simulink model "maglev_linear_model"  (R2021a)
settings: Solver=VariableStepAuto  StartTime=0.0  StopTime=0.2  RelTol=1e-3
settings Model: Creator=user  LastModifiedBy=user

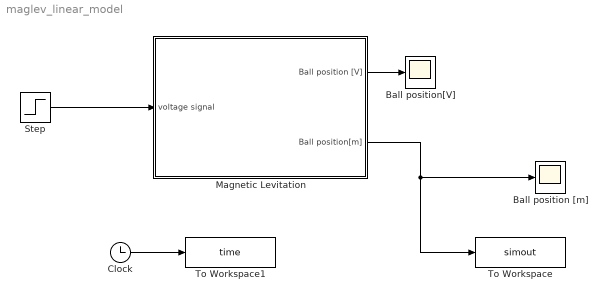
== system maglev_linear_model ==
  Ball position [m] : Scope
  Ball position[V] : Scope
  Clock : Clock
  Magnetic Levitation : Subsystem
  Step : Step  SampleTime=0
  To Workspace : ToWorkspace  VariableName=simout  SampleTime=-1
      settings: Save2DSignal=2-D array (concatenate along first dimension)
  To Workspace1 : ToWorkspace  VariableName=time  SampleTime=0.01
      settings: Save2DSignal=2-D array (concatenate along first dimension)
  wires:
  Step/1 -> Magnetic Levitation/1(voltage signal)
  Magnetic Levitation/2(Ball position[m]) -> To Workspace/1, Ball position [m]/1
  Magnetic Levitation/1(Ball position [V]) -> Ball position[V]/1
  Clock/1 -> To Workspace1/1

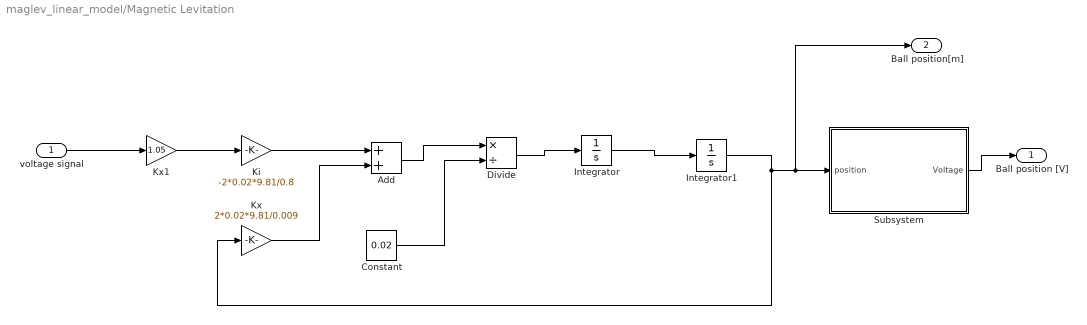
== system maglev_linear_model/Magnetic Levitation ==
  voltage signal : Inport
  Add : Sum
  Constant : Constant  Value=0.02
  Divide : Product  Inputs=*/
  Integrator : Integrator
  Integrator1 : Integrator
  Ki : Gain  Gain=-2*0.02*9.81/0.8
  Kx : Gain  Gain=2*0.02*9.81/0.009
  Kx1 : Gain  Gain=1.05
  Subsystem : Subsystem
  Ball position [V] : Outport  Unit=V
  Ball position[m] : Outport  Port=2  Unit=meter
  wires:
  voltage signal/1 -> Kx1/1
  Kx1/1 -> Ki/1
  Ki/1 -> Add/1
  Kx/1 -> Add/2
  Constant/1 -> Divide/2
  Add/1 -> Divide/1
  Divide/1 -> Integrator/1
  Integrator/1 -> Integrator1/1
  Subsystem/1(Voltage) -> Ball position [V]/1
  Integrator1/1 -> Kx/1, Ball position[m]/1, Subsystem/1(position)

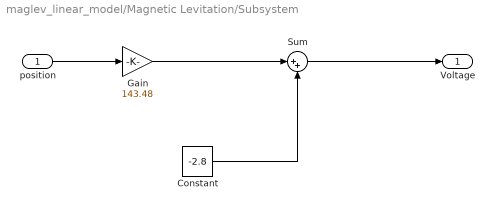
== system maglev_linear_model/Magnetic Levitation/Subsystem ==
  position : Inport
  Constant : Constant  Value=-2.8
  Gain : Gain  Gain=143.48
  Sum : Sum  Inputs=|++
  Voltage : Outport
  wires:
  position/1 -> Gain/1
  Sum/1 -> Voltage/1
  Gain/1 -> Sum/1
  Constant/1 -> Sum/2
